simulink library "csc_gps_piksi_model_lib"  (R2014b)
settings: Solver=ode45  SolverMode=SingleTasking  StartTime=0.0  StopTime=10.0  RelTol=1e-3
undefined symbols (not defined in the file): gps_delay_counts
libraries: util_common_lib x4, simulink x1, util_info_lib x1, csu_pbp_piksi_baseline_packet_lib x1, csu_pep_piksi_earth_fixed_packet_lib x1
settings Model: Creator=eleanor  LastModifiedBy=escrane

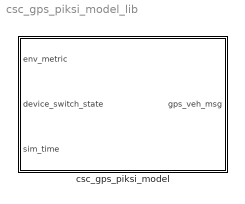
== system csc_gps_piksi_model_lib ==
  csc_gps_piksi_model : Subsystem  SystemSampleTime=0.1

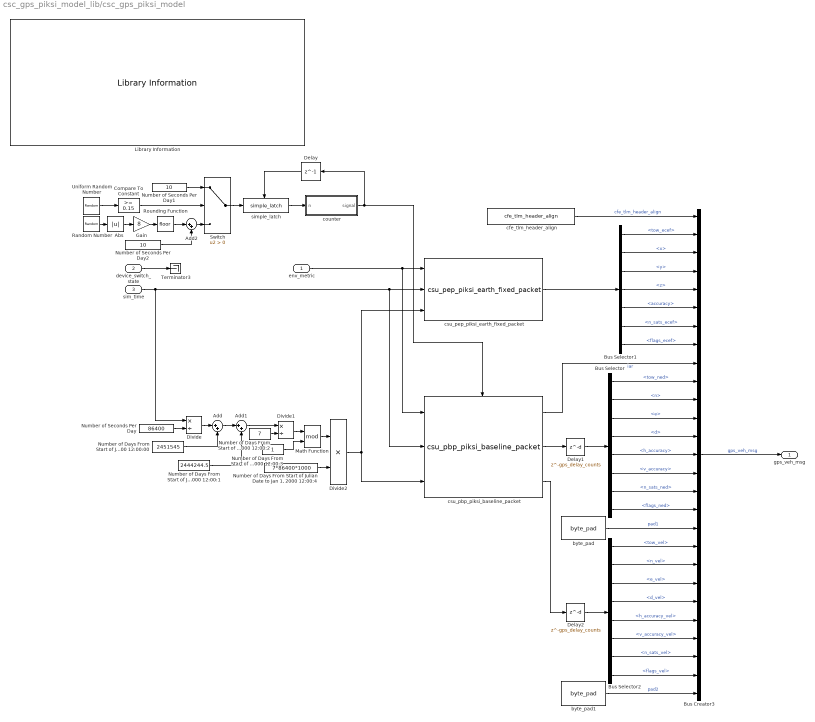
== system csc_gps_piksi_model_lib/csc_gps_piksi_model ==
  env_metric : Inport
  device_switch_state : Inport  Port=2
  sim_time : Inport  Port=3
  Abs : Abs
  Add : Sum  Inputs=|++
  Add1 : Sum  Inputs=|++
  Add2 : Sum  Inputs=|++
  Bus Creator3 : BusCreator  Inputs=27  OutDataTypeStr=Bus: gps_veh_msg  NonVirtualBus=on
  Bus Selector : BusSelector  OutputSignals=tow_ned,n,e,d,h_accuracy,v_accuracy,n_sats_ned,flags_ned
  Bus Selector1 : BusSelector  OutputSignals=tow_ecef,x,y,z,accuracy,n_sats_ecef,flags_ecef
  Bus Selector2 : BusSelector  OutputSignals=tow_vel,n_vel,e_vel,d_vel,h_accuracy_vel,v_accuracy_vel,n_sats_vel,flags_vel
  Compare To Constant : simulink/Logic and Bit Operations/Compare To Constant  relop=>=  const=0.15  OutDataTypeStr=boolean
  Delay : Delay  DelayLength=1  InitialCondition=0
  Delay1 : Delay  DelayLength=gps_delay_counts  InitialCondition=0
  Delay2 : Delay  DelayLength=gps_delay_counts  InitialCondition=0
  Divide : Product  Inputs=*/
  Divide1 : Product  Inputs=*/
  Divide2 : Product  Inputs=**
  Gain : Gain  Gain=8
  Library Information : util_info_lib/Library Information  owner='escrane'
  Math Function : Math  Operator=mod  SaturateOnIntegerOverflow=on
  "Number of Days From Start of Julian Date to Jan 1, 2000 12:00:00" : Constant  Value=2451545
  "Number of Days From Start of Julian Date to Jan 1, 2000 12:00:1" : Constant  Value=2444244.5
  "Number of Days From Start of Julian Date to Jan 1, 2000 12:00:2" : Constant  Value=7
  "Number of Days From Start of Julian Date to Jan 1, 2000 12:00:3" : Constant
  "Number of Days From Start of Julian Date to Jan 1, 2000 12:00:4" : Constant  Value=7*86400*1000
  Number of Seconds Per Day : Constant  Description=|  Value=86400
      | Number of Seconds                   
      | July 4, 2014 22:40:00 UTC           
      | Calculate on Web Site:              
      | www.mbari.org/staff/rich/utccalc.htm
  Number of Seconds Per Day1 : Constant  Description=|  Value=10
      | Number of Seconds                   
      | July 4, 2014 22:40:00 UTC           
      | Calculate on Web Site:              
      | www.mbari.org/staff/rich/utccalc.htm
  Number of Seconds Per Day2 : Constant  Description=|  Value=10
      | Number of Seconds                   
      | July 4, 2014 22:40:00 UTC           
      | Calculate on Web Site:              
      | www.mbari.org/staff/rich/utccalc.htm
  Random Number : RandomNumber  Seed=293  SampleTime=0.01
  Rounding Function : Rounding
  Switch : Switch  Criteria=u2 > Threshold
  Terminator3 : Terminator
  Uniform Random Number : UniformRandomNumber  Minimum=0  Seed=45  SampleTime=0.01
  byte_pad : util_common_lib/byte_pad  n_bytes=2
  byte_pad1 : util_common_lib/byte_pad  n_bytes=2
  cfe_tlm_header_align : util_common_lib/cfe_tlm_header_align
  counter : Subsystem  TreatAsAtomicUnit=on
  csu_pbp_piksi_baseline_packet : csu_pbp_piksi_baseline_packet_lib/csu_pbp_piksi_baseline_packet
  csu_pep_piksi_earth_fixed_packet : csu_pep_piksi_earth_fixed_packet_lib/csu_pep_piksi_earth_fixed_packet
  simple_latch : util_common_lib/simple_latch  SystemSampleTime=-1
  gps_veh_msg : Outport
  wires:
  Switch/1 -> simple_latch/1
  byte_pad1/1 -> Bus Creator3/27  "pad2"
  Bus Selector2/8 -> Bus Creator3/26  "<flags_vel>"
  Bus Selector2/7 -> Bus Creator3/25  "<n_sats_vel>"
  Bus Selector2/6 -> Bus Creator3/24  "<v_accuracy_vel>"
  Bus Selector2/5 -> Bus Creator3/23  "<h_accuracy_vel>"
  Bus Selector2/4 -> Bus Creator3/22  "<d_vel>"
  Bus Selector2/3 -> Bus Creator3/21  "<e_vel>"
  Bus Selector2/2 -> Bus Creator3/20  "<n_vel>"
  Bus Selector2/1 -> Bus Creator3/19  "<tow_vel>"
  Delay2/1 -> Bus Selector2/1
  csu_pbp_piksi_baseline_packet/3 -> Delay2/1
  Rounding Function/1 -> Add2/1
  Gain/1 -> Rounding Function/1
  Compare To Constant/1 -> Switch/2
  Abs/1 -> Gain/1
  Random Number/1 -> Abs/1
  Delay1/1 -> Bus Selector/1
  Delay/1 -> simple_latch/Trigger
  simple_latch/1 -> counter/1(n)
  Number of Seconds Per Day1/1 -> Switch/1
  Add2/1 -> Switch/3
  Number of Seconds Per Day2/1 -> Add2/2
  counter/1(signal) -> Delay/1, csu_pbp_piksi_baseline_packet/Enable
  Uniform Random Number/1 -> Compare To Constant/1
  Bus Selector/7 -> Bus Creator3/16  "<n_sats_ned>"
  Bus Selector/3 -> Bus Creator3/12  "<e>"
  Bus Selector/5 -> Bus Creator3/14  "<h_accuracy>"
  Bus Selector/2 -> Bus Creator3/11  "<n>"
  Bus Selector/4 -> Bus Creator3/13  "<d>"
  Bus Selector/1 -> Bus Creator3/10  "<tow_ned>"
  Bus Selector/8 -> Bus Creator3/17  "<flags_ned>"
  Bus Selector/6 -> Bus Creator3/15  "<v_accuracy>"
  Bus Selector1/6 -> Bus Creator3/7  "<n_sats_ecef>"
  Bus Selector1/3 -> Bus Creator3/4  "<y>"
  Bus Selector1/1 -> Bus Creator3/2  "<tow_ecef>"
  Bus Selector1/7 -> Bus Creator3/8  "<flags_ecef>"
  Bus Selector1/4 -> Bus Creator3/5  "<z>"
  Bus Selector1/2 -> Bus Creator3/3  "<x>"
  Bus Selector1/5 -> Bus Creator3/6  "<accuracy>"
  "Number of Days From Start of Julian Date to Jan 1, 2000 12:00:4"/1 -> Divide2/2
  Math Function/1 -> Divide2/1
  "Number of Days From Start of Julian Date to Jan 1, 2000 12:00:3"/1 -> Math Function/2
  Divide1/1 -> Math Function/1
  "Number of Days From Start of Julian Date to Jan 1, 2000 12:00:2"/1 -> Divide1/2
  Add1/1 -> Divide1/1
  "Number of Days From Start of Julian Date to Jan 1, 2000 12:00:1"/1 -> Add1/2
  Add/1 -> Add1/1
  Number of Seconds Per Day/1 -> Divide/2
  sim_time/1 -> csu_pep_piksi_earth_fixed_packet/2, csu_pbp_piksi_baseline_packet/2, Divide/1
  "Number of Days From Start of Julian Date to Jan 1, 2000 12:00:00"/1 -> Add/2
  Divide/1 -> Add/1
  Divide2/1 -> csu_pep_piksi_earth_fixed_packet/3, csu_pbp_piksi_baseline_packet/3
  csu_pbp_piksi_baseline_packet/1 -> Bus Creator3/9  "iar"
  csu_pbp_piksi_baseline_packet/2 -> Delay1/1
  csu_pep_piksi_earth_fixed_packet/1 -> Bus Selector1/1
  cfe_tlm_header_align/1 -> Bus Creator3/1  "cfe_tlm_header_align"
  env_metric/1 -> csu_pep_piksi_earth_fixed_packet/1, csu_pbp_piksi_baseline_packet/1
  device_switch_state/1 -> Terminator3/1
  Bus Creator3/1 -> gps_veh_msg/1  "gps_veh_msg"
  byte_pad/1 -> Bus Creator3/18  "pad1"

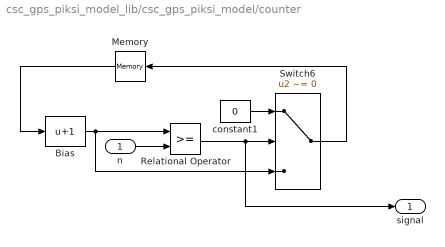
== system csc_gps_piksi_model_lib/csc_gps_piksi_model/counter ==
  n : Inport
  Bias : Bias  Bias=1
  Memory : Memory  X0=20  InheritSampleTime=on
  Relational Operator : RelationalOperator  OutDataTypeStr=boolean
  Switch6 : Switch  Criteria=u2 ~= 0  InputSameDT=on
  constant1 : Constant  Value=0
  signal : Outport
  wires:
  n/1 -> Relational Operator/2
  constant1/1 -> Switch6/1
  Bias/1 -> Relational Operator/1, Switch6/3
  Relational Operator/1 -> Switch6/2, signal/1
  Switch6/1 -> Memory/1
  Memory/1 -> Bias/1
